simulink subsystem "joyToPWM"  (R2025b)
settings: Solver=VariableStepAuto  StartTime=0.0  StopTime=10.0  RelTol=1e-3
undefined symbols (not defined in the file or in its folder): masks, max_thruster_force
settings Model: Creator=kjhaydon  LastModifiedBy=kjhaydon

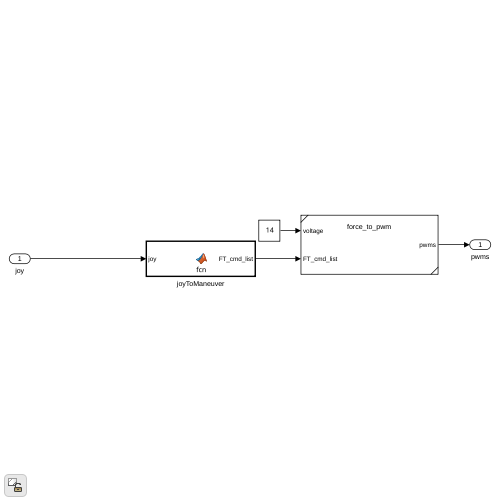
[thumbnail: Simulink's stored preview of the top-level diagram]
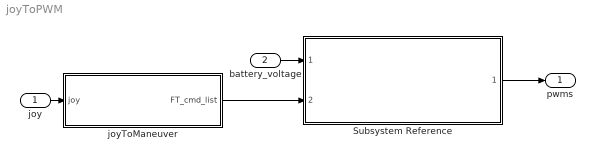
== system joyToPWM ==
  joy : Inport
  battery_voltage : Inport  Port=2
  Subsystem Reference : Subsystem  ReferencedSubsystem=force_to_pwm
  joyToManeuver : MATLAB Function  TreatAsAtomicUnit=on
  pwms : Outport
  wires:
  joyToManeuver/1(FT_cmd_list) -> Subsystem Reference/2
  Subsystem Reference/1 -> pwms/1
  joy/1 -> joyToManeuver/1(joy)
  battery_voltage/1 -> Subsystem Reference/1

== matlab function joyToPWM/joyToManeuver ==
  data: joy input; FT_cmd_list output; masks parameter; max_thruster_force parameter
function FT_cmd_list = fcn(joy,masks, max_thruster_force)

FT_cmd_list = joyToManeuver(joy,masks,max_thruster_force);
